simulink model "DC_AC_standalone"  (R2018a)
settings: Solver=FixedStepDiscrete  StartTime=0.0  StopTime=10.0  RelTol=1e-3
libraries: powerlib x16, simulink x3, powerlib_meascontrol x1
settings Model: Creator=cselzey  LastModifiedBy=cselzey

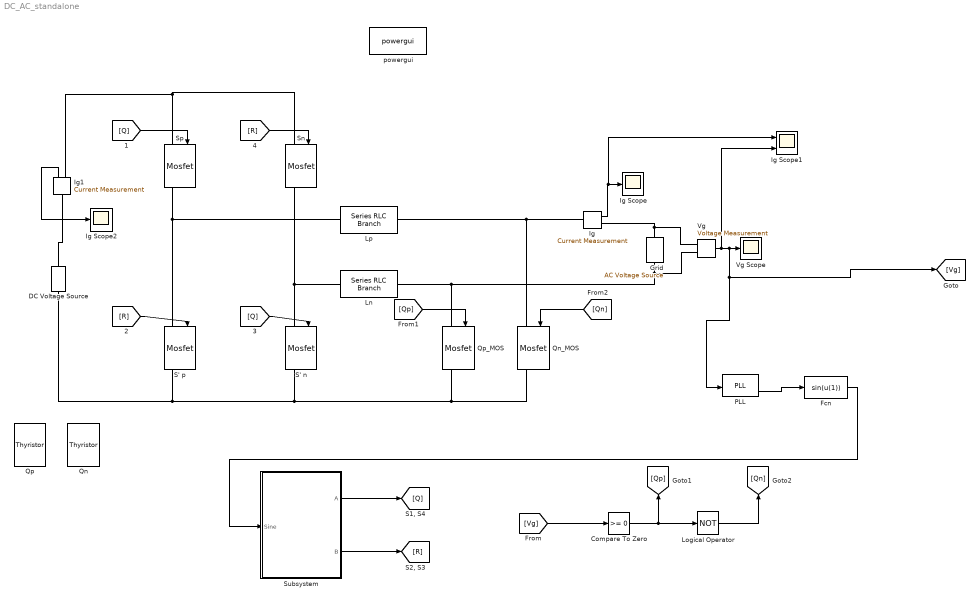
== system DC_AC_standalone ==
  Compare To Zero : simulink/Logic and Bit Operations/Compare To Zero  relop=>=  OutDataTypeStr=boolean
  DC Voltage Source : powerlib/Electrical Sources/DC Voltage Source  Amplitude=350  Measurements=None
  Fcn : Fcn  Expr=sin(u(1))
  Grid : powerlib/Electrical Sources/AC Voltage Source  Amplitude=311.126  Phase=0  Frequency=60  SampleTime=0  Measurements=None  BusType=swing  Pref=10e3  Qref=0  Qmin=-inf  Qmax=+inf
  Ig : powerlib/Measurements/Current Measurement  PhasorSimulation=off  OutputType=Complex  PSBequivalent=0
  Ig Scope : Scope
  Ig Scope1 : Scope  NumInputPorts=2
  Ig Scope2 : Scope
  Ig1 : powerlib/Measurements/Current Measurement  PhasorSimulation=off  OutputType=Complex  PSBequivalent=0
  Ln : powerlib/Elements/Series RLC Branch  LConnTagsString=__new0  RConnTagsString=__new0  BranchType=RL  Resistance=0.000001  Inductance=15e-3  SetiL0=off  InitialCurrent=0  Capacitance=1e-6  Setx0=off  InitialVoltage=0  Measurements=None
  Logical Operator : Logic  Operator=NOT  AllPortsSameDT=off  OutDataTypeStr=boolean
  Lp : powerlib/Elements/Series RLC Branch  LConnTagsString=__new0  RConnTagsString=__new0  BranchType=RL  Resistance=0.000001  Inductance=15e-3  SetiL0=off  InitialCurrent=0  Capacitance=1e-6  Setx0=off  InitialVoltage=0  Measurements=None
  PLL : powerlib_meascontrol/PLL/PLL  Fmin=45  Par_Init=[0, 60]  ParK=[180, 3200, 1]  TcD=1e-4  MaxRateChangeFreq=12  FilterCutOffFreq=25  Ts=1e-6  AGC=on
      settings: SourceProductName=Simscape Power Systems  SourceProductBaseCode=PS
  Qn : powerlib/Power Electronics/Thyristor  Ron=0.001  Lon=0  Vf=0.8  IC=0  Rs=500  Cs=250e-9  Measurements=on
  Qn_MOS : powerlib/Power Electronics/Mosfet  Ron=0.1  Lon=0  Rd=0.01  Vfd=0  IC=0  Rs=1e5  Cs=inf  Measurements=on
  Qp : powerlib/Power Electronics/Thyristor  Ron=0.001  Lon=0  Vf=0.8  IC=0  Rs=500  Cs=250e-9  Measurements=on
  Qp_MOS : powerlib/Power Electronics/Mosfet  Ron=0.1  Lon=0  Rd=0.01  Vfd=0  IC=0  Rs=1e5  Cs=inf  Measurements=on
  S' n : powerlib/Power Electronics/Mosfet  Ron=0.1  Lon=0  Rd=0.01  Vfd=0  IC=0  Rs=1e5  Cs=inf  Measurements=on
  S' p : powerlib/Power Electronics/Mosfet  Ron=0.1  Lon=0  Rd=0.01  Vfd=0  IC=0  Rs=1e5  Cs=inf  Measurements=on
  Sn : powerlib/Power Electronics/Mosfet  Ron=0.1  Lon=0  Rd=0.01  Vfd=0  IC=0  Rs=1e5  Cs=inf  Measurements=on
  Sp : powerlib/Power Electronics/Mosfet  Ron=0.1  Lon=0  Rd=0.01  Vfd=0  IC=0  Rs=1e5  Cs=inf  Measurements=on
  Subsystem : Subsystem
  Vg : powerlib/Measurements/Voltage Measurement  PhasorSimulation=off  OutputType=Complex  PSBequivalent=0
  Vg Scope : Scope
  powergui : powerlib/powergui  Priority=1  SimulationMode=Discrete  SampleTime=50e-6  frequency=60  Iterations=50  frequencyindice=60  Pbase=100e6  ErrMax=1e-4  UnitsV=kV  UnitsW=MW  buscounter=0  FunctionMessages=off  echomessages=off  EnableUseOfTLC=off  CurrentSourceSwitches=off  DisableSnubberDevices=off  DisableRonSwitches=off  DisableVfSwitches=off  DisplayEquations=off  SolverType=Tustin/Backward Euler (TBE)  Interpol=off  ExternalGateDelay=off  methode=off  Ts=100  x0status=blocks  SPID=on  SwTol=0  HookPort=off  RestoreLinks=warning  ResistiveCurrentMeasurement=off  Frange=[0:2:500]  Ylog=off  Xlog=on  ShowGrid=off  save=off  variable=ZData  structure=0  ZoomFFT=off  StartTime=0.0  cycles=1  DisplayStyle=1  fundamental=60  FreqAxis=off  MaxFrequency=1000  frequencyindicesteady=1  RmsSteady=1  display=off
  wires:
  Fcn/1 -> Subsystem/1(Sine)
  [Q] -> S' n/1
  [R] -> S' p/1
  Ig/1 -> Ig Scope1/1, Ig Scope/1
  PLL/2 -> Fcn/1
  Vg/1 -> Ig Scope1/2, [Vg], PLL/1, Vg Scope/1
  [Q] -> Sp/1
  [R] -> Sn/1
  Subsystem/1(A) -> [Q]
  Subsystem/2(B) -> [R]
  Ig1/1 -> Ig Scope2/1
  [Vg] -> Compare To Zero/1
  Compare To Zero/1 -> [Qp], Logical Operator/1
  Logical Operator/1 -> [Qn]
  [Qp] -> Qp_MOS/1
  [Qn] -> Qn_MOS/1
  connections:
  S' p/RConn1 -- S' n/RConn1 -- Qn_MOS/RConn1 -- Qp_MOS/RConn1 -- DC Voltage Source/LConn1
  Sp/RConn1 -- S' p/LConn1 -- Lp/LConn1
  Grid/RConn1 -- Vg/LConn1 -- Ig/RConn1
  S' n/LConn1 -- Sn/RConn1 -- Ln/LConn1
  Grid/LConn1 -- Qp_MOS/LConn1 -- Ln/RConn1 -- Vg/LConn2
  Ig/LConn1 -- Qn_MOS/LConn1 -- Lp/RConn1
  Sn/LConn1 -- Ig1/RConn1 -- Sp/LConn1
  Ig1/LConn1 -- DC Voltage Source/RConn1

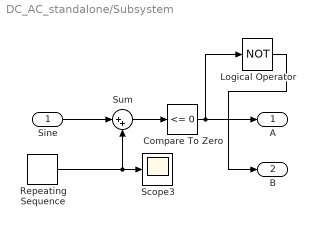
== system DC_AC_standalone/Subsystem ==
  Sine : Inport
  Compare To Zero : simulink/Logic and Bit Operations/Compare To Zero  relop=<=  OutDataTypeStr=boolean
  Logical Operator : Logic  Operator=NOT  AllPortsSameDT=off  OutDataTypeStr=boolean
  Repeating Sequence : simulink/Sources/Repeating Sequence  rep_seq_t=[0 1/(4*16000) 3/(4*16000) 1/16000]  rep_seq_y=[0 1 -1 0]
  Scope3 : Scope
  Sum : Sum  Inputs=|++
  A : Outport
  B : Outport  Port=2
  wires:
  Compare To Zero/1 -> A/1, Logical Operator/1
  Logical Operator/1 -> B/1
  Sum/1 -> Compare To Zero/1
  Repeating Sequence/1 -> Scope3/1, Sum/2
  Sine/1 -> Sum/1
